simulink model "PubIfDecisionVSM_ACC"  (R2020b)
settings: Solver=FixedStepAuto  StartTime=0.0  StopTime=Inf  RelTol=1e-3
PostLoadFcn:
  | if any(exist('dsrtsu_mdlpostloadfcn', 'file') ~= 0), dsrtsu_mdlpostloadfcn('Execute', bdroot); end
InitFcn:
  | , if any(exist('dsmpb_private', 'file') ~= 0), dsmpb_private('dsmpb_mdlclblib', 'Init', bdroot); end,
PreSaveFcn:
  | , if any(exist('dsmpb_private', 'file') ~= 0), dsmpb_private('dsmpb_mdlclblib', 'PreSave', bdroot); end,
CloseFcn:
  | , if any(exist('dsmpb_private', 'file') ~= 0), dsmpb_private('dsmpb_mdlclblib', 'Close', bdroot); end,
settings Model: DataDictionary=HWA_DDs.sldd  RTICANMMDATA=struct('GeneralSetupData',struct('modelroot','C:\Users\GW00208968\Desktop\newhwa\Adas\VSM\ACC','generalsettings',struct('filesettings',struct('destfolder',struct('Name','RTICANMM_FILES','Check',1),'buildfolder',struct('Name','.','Check',1),'AbsDestfolder',struct('Name','C:\Users\GW00208968\Desktop\newhwa\Adas\VSM\ACC\RTICANMM_FILES'),'AbsBuildfolder',struct('Name','C:\Users\GW00208968\Desktop\newhwa\Adas\VSM\ACC'))),'options',struct('addpaths',1,'rmpaths',1,'addtrcexclusion',false,'cannavigator',struct('checkmonitoring',0),'show_usrtrc',0,'use_usrtrc',0),'advanced',struct('options',ones(1,100)),'MPSetup',{{}},'RTI',struct('Type','DSRT','Ver','4.2','Date','02-Nov-2019'),'modelname','PubIfDecisionVSM_ACC','block','PubIfDecisionVSM_ACC'))  DSRTSU_INTERNAL_RTIFPGA=150  Creator=GW00180895  LastModifiedBy=GW00208968
settings OptimizationCC: BlockReduction=off  ConditionallyExecuteInputs=off  OptimizeBlockIOStorage=off  BufferReuse=off  GlobalBufferReuse=off  ExpressionFolding=off  LocalBlockOutputs=off  OptimizeDataStoreBuffers=off  BusAssignmentInplaceUpdate=off
settings DebuggingCC: TasksWithSamePriorityMsg=none
settings HardwareCC: ProdBitPerPointer=32  ProdBitPerSizeT=32  ProdBitPerPtrDiffT=32  ProdLargestAtomicInteger=Integer  ProdWordSize=32  ProdHWDeviceType=Custom Processor->Custom
settings ModelReferenceCC: UpdateModelReferenceTargets=IfOutOfDate  EnableParallelModelReferenceBuilds=on  ModelReferenceNumInstancesAllowed=Single
settings SFSimCC: MATLABDynamicMemAlloc=off
settings RTWCC: Description=dSPACE Run-Time Target (for VEOS on Windows and ConfigurationDesk)  SystemTargetFile=dsrt.tlc  GenCodeOnly=on  MakeCommand=make_dsrt  TemplateMakefile=dsrt_default_tmf  RTWVerbose=off
settings CodeAppCC: MaxIdLength=128
settings STFCustomTargetCC: TargetLangStandard=C99 (ISO)  ParMdlRefBuildCompliant=on  ConcurrentExecutionCompliant=off  CPPClassGenCompliant=off  GRTInterface=off  SystemTargetFile=dsrt.tlc
settings GRTTargetCC: CompOptLevelCompliant=off  ConcurrentExecutionCompliant=off  CombineOutputUpdateFcns=off  MatFileLogging=off  CPPClassGenCompliant=off  UseToolchainInfoCompliant=off

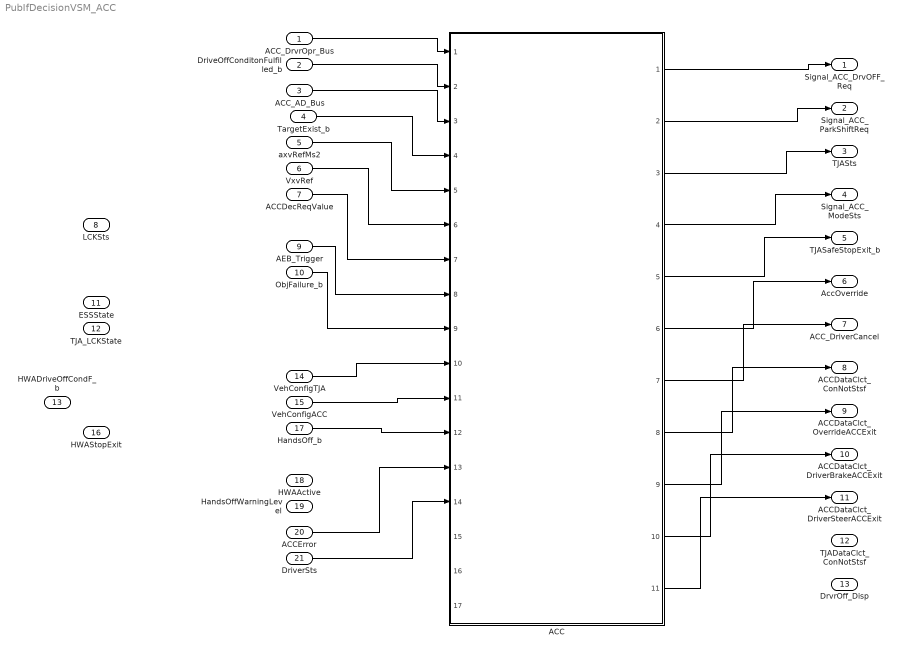
== system PubIfDecisionVSM_ACC ==
  ACC_DrvrOpr_Bus : Inport  OutDataTypeStr=Bus: ACC_DrvrOpr_Bus
  DriveOffConditonFulfilled_b : Inport  Port=2  OutDataTypeStr=boolean
  ACC_AD_Bus : Inport  Port=3  OutDataTypeStr=Bus: ACC_AD_Bus
  TargetExist_b : Inport  Port=4  OutDataTypeStr=boolean
  axvRefMs2 : Inport  Port=5  OutDataTypeStr=single
  VxvRef : Inport  Port=6  OutDataTypeStr=single
  ACCDecReqValue : Inport  Port=7  OutDataTypeStr=single
  LCKSts : Inport  Port=8  OutDataTypeStr=Enum: LCK_STATE
  AEB_Trigger : Inport  Port=9  OutDataTypeStr=boolean
  ObjFailure_b : Inport  Port=10  OutDataTypeStr=boolean
  ESSState : Inport  Port=11  OutDataTypeStr=uint8
  TJA_LCKState : Inport  Port=12  OutDataTypeStr=Enum: LCK_STATE
  HWADriveOffCondF_b : Inport  Port=13  OutDataTypeStr=boolean
  VehConfigTJA : Inport  Port=14  OutDataTypeStr=boolean
  VehConfigACC : Inport  Port=15  OutDataTypeStr=boolean
  HWAStopExit : Inport  Port=16  OutDataTypeStr=boolean
  HandsOff_b : Inport  Port=17  OutDataTypeStr=boolean
  HWAActive : Inport  Port=18  OutDataTypeStr=boolean
  HandsOffWarningLevel : Inport  Port=19  OutDataTypeStr=uint8
  ACCError : Inport  Port=20  OutDataTypeStr=uint8
  DriverSts : Inport  Port=21  OutDataTypeStr=uint8
  ACC : Subsystem  ReferencedSubsystem=PvtSubSys_VSM_ACC
  Signal_ACC_DrvOFF_Req : Outport
  Signal_ACC_ParkShiftReq : Outport  Port=2
  TJASts : Outport  Port=3
  Signal_ACC_ModeSts : Outport  Port=4
  TJASafeStopExit_b : Outport  Port=5
  AccOverride : Outport  Port=6
  ACC_DriverCancel : Outport  Port=7
  ACCDataClct_ConNotStsf : Outport  Port=8
  ACCDataClct_OverrideACCExit : Outport  Port=9
  ACCDataClct_DriverBrakeACCExit : Outport  Port=10
  ACCDataClct_DriverSteerACCExit : Outport  Port=11
  TJADataClct_ConNotStsf : Outport  Port=12
  DrvrOff_Disp : Outport  Port=13
  wires:
  ACC_DrvrOpr_Bus/1 -> ACC/1
  DriveOffConditonFulfilled_b/1 -> ACC/2
  ACC_AD_Bus/1 -> ACC/3
  ACC/1 -> Signal_ACC_DrvOFF_Req/1
  ACC/2 -> Signal_ACC_ParkShiftReq/1
  ACC/3 -> TJASts/1
  ACC/4 -> Signal_ACC_ModeSts/1
  ACC/5 -> TJASafeStopExit_b/1
  ACC/6 -> AccOverride/1
  ACC/7 -> ACC_DriverCancel/1
  ACC/8 -> ACCDataClct_ConNotStsf/1
  ACC/9 -> ACCDataClct_OverrideACCExit/1
  ACC/10 -> ACCDataClct_DriverBrakeACCExit/1
  ACC/11 -> ACCDataClct_DriverSteerACCExit/1
  ? -> TJADataClct_ConNotStsf/1
  ? -> DrvrOff_Disp/1
  TargetExist_b/1 -> ACC/4
  axvRefMs2/1 -> ACC/5
  VxvRef/1 -> ACC/6
  ACCDecReqValue/1 -> ACC/7
  AEB_Trigger/1 -> ACC/8
  ObjFailure_b/1 -> ACC/9
  VehConfigACC/1 -> ACC/11
  VehConfigTJA/1 -> ACC/10
  HandsOff_b/1 -> ACC/12
  DriverSts/1 -> ACC/14
  ACCError/1 -> ACC/13
